simulink model "quadrotor_sim"  (Simulink 7.7)
settings: Solver=FixedStepDiscrete  StartTime=0.0  StopTime=120  FixedStep=1/50  RelTol=1e-3
undefined symbols (not defined in the file): alpha_IERA_IELA_IELA, bus_Environment, Kutta, R_IERA_RA_RA, Runge
libraries: UAVdesign_net x8
settings Model: Creator=Emanuel  LastModifiedBy=Emanuel
settings SFSimCC: SimCustomHeaderCode="#include \"cd_signals.h\""  SimUserSources=cd_signals.c

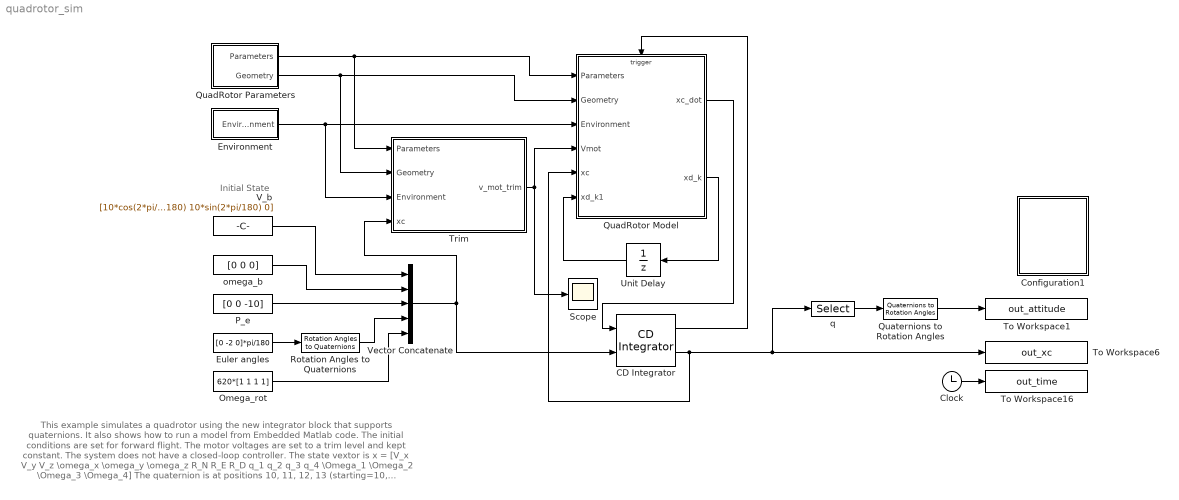
== system quadrotor_sim ==
  note: This example simulates a quadrotor using the new integrator block that supports quaternions. It also shows how to run a model from Embedded Matlab code.
      | The initial conditions are set for forward flight. The motor voltages are set to a trim level and kept constant. The system does not have a closed-loop controller.
      | The state vextor is x = [V_x V_y V_z   \omega_x \omega_y \omega_z    R_N R_E R_D    q_1 q_2 q_3 q_4    \Omega_1 \Omega_2 \Omega_3 \Omega_4]
      | The quaternion is at positions 10, 11, 12, 13 (starting=10, ending=13)
      | \Omega^{\bullet} is at positions 4, 5, 6
  note: Initial State
  CD Integrator : UAVdesign_net/Utilities/Continuous/CD Integrator  algorithm=Runge-Kutta  param_source=Discrete steps of the model  initial_time=0  final_time=10  reset_type=None  x0_source=External  x0=0  output_time=off  limit_output=off  upper_sat=inf  lower_sat=-inf  q_index=[10 13]  omega_dot_index=[4 6]  sample_time=-1
  Clock : Clock
  Configuration1 : Subsystem
      settings: OpenFcn=graphs_quadrotor_sim;
      mask Display: disp('Double-click\nto display\nthe\ngraphs')
  Environment : Subsystem  InitFcn=bus_Environment;
  Euler angles : Constant  Value=[0 -2 0]*pi/180
  Omega_rot : Constant  Value=620*[1 1 1 1]
  P_e : Constant  Value=[0 0 -10]
  QuadRotor Model : Subsystem
  QuadRotor Parameters : Subsystem  InitFcn=|  mask(HelicopterParameters){}
      | bus_PropellerParameters;    
      | bus_ElectricMotorParameters;
      | bus_GeometryParameters;     
      | bus_FuselageParameters;
      mask help:
      | Parameters for a helicopter.
      | Geometry, rotors, fuselage, fins.
      mask init:
      | set_param(gcb, 'LinkStatus', 'none');
      settings: OpenFcn=gui_QuadRotorParameters( 'Block', [get_param(gcb, 'Parent') '/' get_param(gcb, 'Name')]);
      mask Display:
      | port_label('output', 1, 'Parameters')
      | port_label('output', 2, 'Geometry')
  Quaternions to Rotation Angles : UAVdesign_net/Utilities/Axes/Quaternions to Rotation Angles  SystemSampleTime=-1
  Rotation Angles to Quaternions : UAVdesign_net/Utilities/Axes/Rotation Angles to Quaternions  SystemSampleTime=-1
  Scope : Scope
      settings: YMin=7.37  YMax=7.415
  To Workspace1 : ToWorkspace  VariableName=out_attitude  SampleTime=-1  SaveFormat=Array
  To Workspace16 : ToWorkspace  VariableName=out_time  SampleTime=-1  SaveFormat=Array
  To Workspace6 : ToWorkspace  VariableName=out_xc  SampleTime=-1  SaveFormat=Array
  Trim : Subsystem
  Unit Delay : UnitDelay  X0=[zeros(12,1); 1;1;1;1; zeros(7,1)]  SampleTime=-1
  V_b : Constant  Value=[10*cos(2*pi/180) 10*sin(2*pi/180) 0]
  Vector Concatenate : Concatenate  NumInputs=5  Mode=Vector
  omega_b : Constant  Value=[0 0 0]
  q : Selector  InputPortWidth=17  IndexOptions=Index vector (dialog)  Indices=[10:13]  OutputSizes=1
  wires:
  QuadRotor Model/2(xd_k) -> Unit Delay/1
  Unit Delay/1 -> QuadRotor Model/6(xd_k1)
  QuadRotor Model/1(xc_dot) -> CD Integrator/1
  CD Integrator/1 -> QuadRotor Model/Trigger
  CD Integrator/2 -> QuadRotor Model/5(xc), To Workspace6/1, q/1
  QuadRotor Parameters/1(Parameters) -> QuadRotor Model/1(Parameters), Trim/1(Parameters)
  QuadRotor Parameters/2(Geometry) -> QuadRotor Model/2(Geometry), Trim/2(Geometry)
  Environment/1(Environment) -> QuadRotor Model/3(Environment), Trim/3(Environment)
  Trim/1(v_mot_trim) -> QuadRotor Model/4(Vmot), Scope/1
  Clock/1 -> To Workspace16/1
  q/1 -> Quaternions to Rotation Angles/1
  Quaternions to Rotation Angles/1 -> To Workspace1/1
  Euler angles/1 -> Rotation Angles to Quaternions/1
  V_b/1 -> Vector Concatenate/1
  omega_b/1 -> Vector Concatenate/2
  P_e/1 -> Vector Concatenate/3
  Rotation Angles to Quaternions/1 -> Vector Concatenate/4
  Omega_rot/1 -> Vector Concatenate/5
  Vector Concatenate/1 -> CD Integrator/2, Trim/4(xc)

== system quadrotor_sim/Configuration1 ==

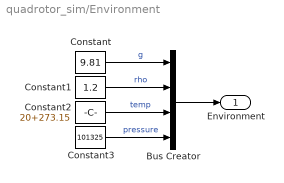
== system quadrotor_sim/Environment ==
  Bus Creator : BusCreator  NonVirtualBus=on
  Constant : Constant  Value=9.81
  Constant1 : Constant  Value=1.2
  Constant2 : Constant  Value=20+273.15
  Constant3 : Constant  Value=101325
  Environment : Outport
  wires:
  Constant3/1 -> Bus Creator/4  "pressure"
  Constant2/1 -> Bus Creator/3  "temp"
  Constant1/1 -> Bus Creator/2  "rho"
  Constant/1 -> Bus Creator/1  "g"
  Bus Creator/1 -> Environment/1

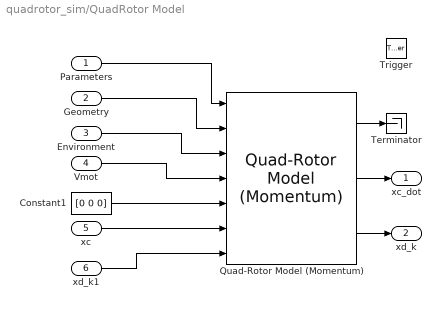
== system quadrotor_sim/QuadRotor Model ==
  Parameters : Inport
  Geometry : Inport  Port=2
  Environment : Inport  Port=3
  Vmot : Inport  Port=4
  xc : Inport  Port=5
  xd_k1 : Inport  Port=6
  Trigger : TriggerPort  TriggerType=function-call
  Constant1 : Constant  Value=[0 0 0]
  Quad-Rotor Model (Momentum) : UAVdesign_net/Vehicle Models/Quad-Rotor Model (Momentum)  SystemSampleTime=-1
  Terminator : Terminator
  xc_dot : Outport
  xd_k : Outport  Port=2
  wires:
  Geometry/1 -> Quad-Rotor Model (Momentum)/2
  xd_k1/1 -> Quad-Rotor Model (Momentum)/7
  xc/1 -> Quad-Rotor Model (Momentum)/6
  Environment/1 -> Quad-Rotor Model (Momentum)/3
  Parameters/1 -> Quad-Rotor Model (Momentum)/1
  Quad-Rotor Model (Momentum)/1 -> Terminator/1
  Constant1/1 -> Quad-Rotor Model (Momentum)/5
  Vmot/1 -> Quad-Rotor Model (Momentum)/4
  Quad-Rotor Model (Momentum)/3 -> xd_k/1
  Quad-Rotor Model (Momentum)/2 -> xc_dot/1

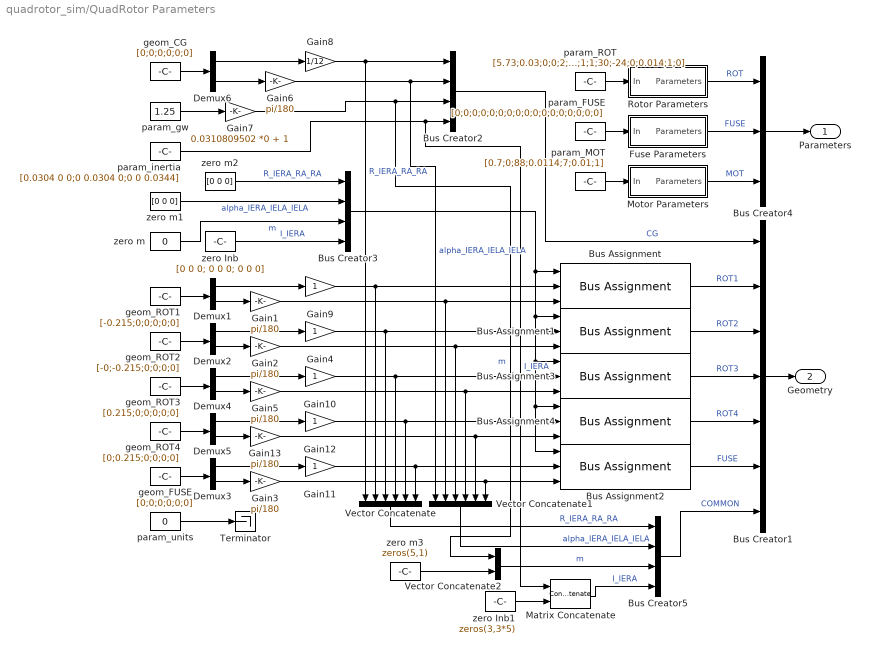
== system quadrotor_sim/QuadRotor Parameters ==
  Bus Assignment{,1..4} (5 alike) : BusAssignment  AssignedSignals=R_IERA_RA_RA,alpha_IERA_IELA_IELA
  Bus Creator1 : BusCreator  Inputs=7
  Bus Creator2 : BusCreator
  Bus Creator3 : BusCreator
  Bus Creator4 : BusCreator  Inputs=3
  Bus Creator5 : BusCreator
  Demux{1..6} (6 alike) : Demux  Outputs=2
  Fuse Parameters : Subsystem
  Gain{1..3,5..6,13} (6 alike) : Gain  Gain=pi/180
  Gain{4,9..12} (5 alike) : Gain
  Gain7 : Gain  Gain=0.0310809502 *0 + 1
  Gain8 : Gain  Gain=1/12
  Matrix Concatenate : Concatenate  Mode=Multidimensional array  ConcatenateDimension=2
  Motor Parameters : Subsystem
  Rotor Parameters : Subsystem
  Terminator : Terminator
  Vector Concatenate : Concatenate  NumInputs=6  Mode=Vector
  Vector Concatenate1 : Concatenate  NumInputs=6  Mode=Vector
  Vector Concatenate2 : Concatenate  Mode=Vector
  geom_CG : Constant  Value=[0;0;0;0;0;0]
  geom_FUSE : Constant  Value=[0;0;0;0;0;0]
  geom_ROT1 : Constant  Value=[-0.215;0;0;0;0;0]
  geom_ROT2 : Constant  Value=[-0;-0.215;0;0;0;0]
  geom_ROT3 : Constant  Value=[0.215;0;0;0;0;0]
  geom_ROT4 : Constant  Value=[0;0.215;0;0;0;0]
  param_FUSE : Constant  Value=[0;0;0;0;0;0;0;0;0;0;0;0;0;0;0;0;0]
  param_MOT : Constant  Value=[0.7;0;88;0.0114;7;0.01;1]
  param_ROT : Constant  Value=[5.73;0.03;0;0;2;0.127;0.016;0.95;1;1;30;-24;0;0.014;1;0]
  param_gw : Constant  Value=1.25
  param_inertia : Constant  Value=[0.0304 0 0;0 0.0304 0;0 0 0.0344]
  param_units : Constant  Value=0
  zero Inb : Constant  Value=[0 0 0; 0 0 0; 0 0 0]
  zero Inb1 : Constant  Value=zeros(3,3*5)
  zero m : Constant  Value=0
  zero m1 : Constant  Value=[0 0 0]
  zero m2 : Constant  Value=[0 0 0]
  zero m3 : Constant  Value=zeros(5,1)
  Parameters : Outport
  Geometry : Outport  Port=2
  wires:
  zero m3/1 -> Vector Concatenate2/2
  Vector Concatenate2/1 -> Bus Creator5/3  "m"
  Bus Creator1/1 -> Geometry/1
  Demux6/1 -> Gain8/1
  Demux6/2 -> Gain6/1
  param_gw/1 -> Gain7/1
  Demux1/1 -> Gain9/1
  Demux1/2 -> Gain1/1
  geom_ROT1/1 -> Demux1/1
  Demux3/1 -> Gain11/1
  Demux3/2 -> Gain3/1
  geom_FUSE/1 -> Demux3/1
  geom_CG/1 -> Demux6/1
  Bus Creator3/1 -> Bus Assignment/1, Bus Assignment1/1, Bus Assignment3/1, Bus Assignment2/1, Bus Assignment4/1
  Bus Creator4/1 -> Parameters/1
  param_ROT/1 -> Rotor Parameters/1(In)
  param_FUSE/1 -> Fuse Parameters/1(In)
  Gain1/1 -> Bus Assignment/3, Vector Concatenate1/2
  Gain3/1 -> Bus Assignment2/3, Vector Concatenate1/6
  Gain11/1 -> Bus Assignment2/2, Vector Concatenate/6
  Bus Assignment2/1 -> Bus Creator1/6  "FUSE"
  Bus Assignment/1 -> Bus Creator1/2  "ROT1"
  Bus Creator2/1 -> Bus Creator1/1  "CG"
  zero m2/1 -> Bus Creator3/1  "R_IERA_RA_RA"
  zero m1/1 -> Bus Creator3/2  "alpha_IERA_IELA_IELA"
  param_units/1 -> Terminator/1
  Rotor Parameters/1(Parameters) -> Bus Creator4/1  "ROT"
  Fuse Parameters/1(Parameters) -> Bus Creator4/2  "FUSE"
  Gain8/1 -> Bus Creator2/1, Vector Concatenate/1  "R_IERA_RA_RA"
  Gain6/1 -> Bus Creator2/2, Vector Concatenate1/1  "alpha_IERA_IELA_IELA"
  zero Inb/1 -> Bus Creator3/4  "I_IERA"
  zero m/1 -> Bus Creator3/3  "m"
  Gain7/1 -> Vector Concatenate2/1, Bus Creator2/3  "m"
  param_inertia/1 -> Bus Creator2/4, Matrix Concatenate/1  "I_IERA"
  Demux2/1 -> Gain4/1
  Demux2/2 -> Gain2/1
  Gain2/1 -> Bus Assignment1/3, Vector Concatenate1/3
  Gain4/1 -> Bus Assignment1/2, Vector Concatenate/3
  geom_ROT2/1 -> Demux2/1
  Gain9/1 -> Bus Assignment/2, Vector Concatenate/2
  Demux4/1 -> Gain10/1
  Demux4/2 -> Gain5/1
  Gain5/1 -> Bus Assignment3/3, Vector Concatenate1/4
  Gain10/1 -> Bus Assignment3/2, Vector Concatenate/4
  geom_ROT3/1 -> Demux4/1
  Demux5/1 -> Gain12/1
  Demux5/2 -> Gain13/1
  Gain13/1 -> Bus Assignment4/3, Vector Concatenate1/5
  Gain12/1 -> Bus Assignment4/2, Vector Concatenate/5
  geom_ROT4/1 -> Demux5/1
  Bus Assignment1/1 -> Bus Creator1/3  "ROT2"
  Bus Assignment3/1 -> Bus Creator1/4  "ROT3"
  Bus Assignment4/1 -> Bus Creator1/5  "ROT4"
  Bus Creator5/1 -> Bus Creator1/7  "COMMON"
  Vector Concatenate1/1 -> Bus Creator5/2  "alpha_IERA_IELA_IELA"
  Matrix Concatenate/1 -> Bus Creator5/4  "I_IERA"
  Vector Concatenate/1 -> Bus Creator5/1  "R_IERA_RA_RA"
  zero Inb1/1 -> Matrix Concatenate/2
  param_MOT/1 -> Motor Parameters/1(In)
  Motor Parameters/1(Parameters) -> Bus Creator4/3  "MOT"

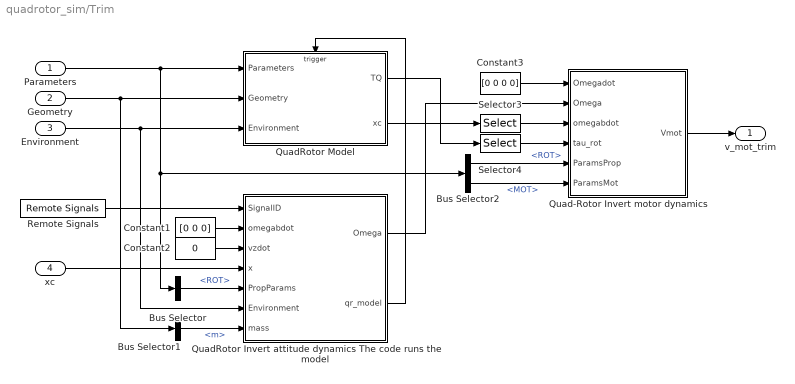
== system quadrotor_sim/Trim ==
  Parameters : Inport
  Geometry : Inport  Port=2
  Environment : Inport  Port=3
  xc : Inport  Port=4
  Bus Selector : BusSelector  OutputSignals=ROT
  Bus Selector1 : BusSelector  OutputSignals=CG.m
  Bus Selector2 : BusSelector  OutputSignals=ROT,MOT
  Constant1 : Constant  Value=[0 0 0]
  Constant2 : Constant  Value=0
  Constant3 : Constant  Value=[0 0 0 0]
  Quad-Rotor Invert motor dynamics : Stateflow chart  TreatAsAtomicUnit=on
  QuadRotor Invert attitude dynamics The code runs the model : Stateflow chart  TreatAsAtomicUnit=on
  QuadRotor Model : Subsystem
  Remote Signals : UAVdesign_net/Utilities/Continuous/Remote Signals  block_name='InvFM_Omega'  op_mode=Generate the signals ID  port_vector=[17 5*4+3]  sample_time=-1
  Selector3 : Selector  InputPortWidth=17  IndexOptions=Index vector (dialog)  Indices=[4:6]  OutputSizes=1
  Selector4 : Selector  InputPortWidth=8  IndexOptions=Index vector (dialog)  Indices=[2 4 6 8]  OutputSizes=1
  v_mot_trim : Outport
  wires:
  Parameters/1 -> QuadRotor Model/1(Parameters), Bus Selector/1, Bus Selector2/1
  Geometry/1 -> QuadRotor Model/2(Geometry), Bus Selector1/1
  Environment/1 -> QuadRotor Model/3(Environment), QuadRotor Invert attitude dynamics The code runs the model/6(Environment)
  Remote Signals/1 -> QuadRotor Invert attitude dynamics The code runs the model/1(SignalID)
  QuadRotor Invert attitude dynamics The code runs the model/2(qr_model) -> QuadRotor Model/Trigger
  xc/1 -> QuadRotor Invert attitude dynamics The code runs the model/4(x)
  Bus Selector/1 -> QuadRotor Invert attitude dynamics The code runs the model/5(PropParams)  "<ROT>"
  Bus Selector1/1 -> QuadRotor Invert attitude dynamics The code runs the model/7(mass)  "<m>"
  Constant1/1 -> QuadRotor Invert attitude dynamics The code runs the model/2(omegabdot)
  Constant2/1 -> QuadRotor Invert attitude dynamics The code runs the model/3(vzdot)
  Selector3/1 -> Quad-Rotor Invert motor dynamics/3(omegabdot)
  Selector4/1 -> Quad-Rotor Invert motor dynamics/4(tau_rot)
  Bus Selector2/1 -> Quad-Rotor Invert motor dynamics/5(ParamsProp)  "<ROT>"
  Bus Selector2/2 -> Quad-Rotor Invert motor dynamics/6(ParamsMot)  "<MOT>"
  Constant3/1 -> Quad-Rotor Invert motor dynamics/1(Omegadot)
  QuadRotor Invert attitude dynamics The code runs the model/1(Omega) -> Quad-Rotor Invert motor dynamics/2(Omega)
  QuadRotor Model/1(TQ) -> Selector4/1
  QuadRotor Model/2(xc) -> Selector3/1
  Quad-Rotor Invert motor dynamics/1(Vmot) -> v_mot_trim/1

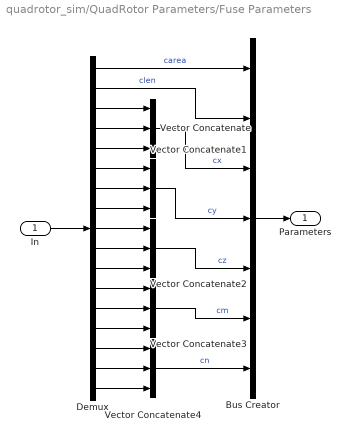
== system quadrotor_sim/QuadRotor Parameters/Fuse Parameters ==
  In : Inport
  Bus Creator : BusCreator  Inputs=7  OutDataTypeStr=Bus: FuselageParameters  NonVirtualBus=on
  Demux : Demux  Outputs=17
  Vector Concatenate{,1..4} (5 alike) : Concatenate  NumInputs=3  Mode=Vector
  Parameters : Outport  OutDataTypeStr=Bus: FuselageParameters
  wires:
  Demux/1 -> Bus Creator/1  "carea"
  Bus Creator/1 -> Parameters/1
  In/1 -> Demux/1
  Demux/2 -> Bus Creator/2  "clen"
  Demux/3 -> Vector Concatenate/1
  Demux/4 -> Vector Concatenate/2
  Demux/5 -> Vector Concatenate/3
  Vector Concatenate/1 -> Bus Creator/3  "cx"
  Demux/6 -> Vector Concatenate1/1
  Demux/7 -> Vector Concatenate1/2
  Demux/8 -> Vector Concatenate1/3
  Vector Concatenate1/1 -> Bus Creator/4  "cy"
  Demux/9 -> Vector Concatenate2/1
  Demux/10 -> Vector Concatenate2/2
  Demux/11 -> Vector Concatenate2/3
  Vector Concatenate2/1 -> Bus Creator/5  "cz"
  Demux/12 -> Vector Concatenate3/1
  Demux/13 -> Vector Concatenate3/2
  Demux/14 -> Vector Concatenate3/3
  Demux/15 -> Vector Concatenate4/1
  Demux/16 -> Vector Concatenate4/2
  Demux/17 -> Vector Concatenate4/3
  Vector Concatenate3/1 -> Bus Creator/6  "cm"
  Vector Concatenate4/1 -> Bus Creator/7  "cn"

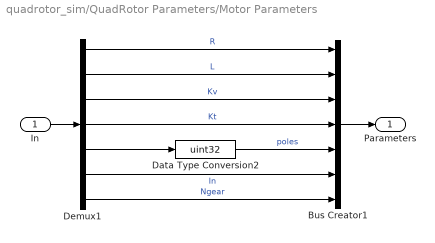
== system quadrotor_sim/QuadRotor Parameters/Motor Parameters ==
  In : Inport
  Bus Creator1 : BusCreator  Inputs=7  NonVirtualBus=on
  Data Type Conversion2 : DataTypeConversion  OutDataTypeStr=uint32  RndMeth=Nearest
  Demux1 : Demux  Outputs=7
  Parameters : Outport
  wires:
  In/1 -> Demux1/1
  Bus Creator1/1 -> Parameters/1
  Demux1/1 -> Bus Creator1/1  "R"
  Demux1/2 -> Bus Creator1/2  "L"
  Demux1/3 -> Bus Creator1/3  "Kv"
  Demux1/4 -> Bus Creator1/4  "Kt"
  Demux1/5 -> Data Type Conversion2/1
  Data Type Conversion2/1 -> Bus Creator1/5  "poles"
  Demux1/6 -> Bus Creator1/6  "In"
  Demux1/7 -> Bus Creator1/7  "Ngear"

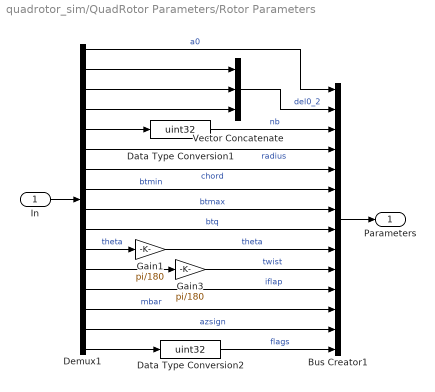
== system quadrotor_sim/QuadRotor Parameters/Rotor Parameters ==
  In : Inport
  Bus Creator1 : BusCreator  Inputs=14  NonVirtualBus=on
  Data Type Conversion1 : DataTypeConversion  OutDataTypeStr=uint32  RndMeth=Nearest
  Data Type Conversion2 : DataTypeConversion  OutDataTypeStr=uint32  RndMeth=Nearest
  Demux1 : Demux  Outputs=16
  Gain1 : Gain  Gain=pi/180
  Gain3 : Gain  Gain=pi/180
  Vector Concatenate : Concatenate  NumInputs=3  Mode=Vector
  Parameters : Outport
  wires:
  Demux1/15 -> Bus Creator1/13  "azsign"
  Demux1/14 -> Bus Creator1/12  "mbar"
  Demux1/13 -> Bus Creator1/11  "iflap"
  Demux1/9 -> Bus Creator1/7  "btmax"
  Demux1/1 -> Bus Creator1/1  "a0"
  Bus Creator1/1 -> Parameters/1
  Demux1/4 -> Vector Concatenate/3
  Demux1/3 -> Vector Concatenate/2
  Demux1/2 -> Vector Concatenate/1
  In/1 -> Demux1/1
  Data Type Conversion1/1 -> Bus Creator1/3  "nb"
  Demux1/5 -> Data Type Conversion1/1
  Demux1/6 -> Bus Creator1/4  "radius"
  Demux1/7 -> Bus Creator1/5  "chord"
  Demux1/8 -> Bus Creator1/6  "btmin"
  Demux1/12 -> Gain3/1
  Demux1/10 -> Bus Creator1/8  "btq"
  Demux1/11 -> Gain1/1  "theta"
  Gain1/1 -> Bus Creator1/9  "theta"
  Vector Concatenate/1 -> Bus Creator1/2  "del0_2"
  Gain3/1 -> Bus Creator1/10  "twist"
  Demux1/16 -> Data Type Conversion2/1
  Data Type Conversion2/1 -> Bus Creator1/14  "flags"

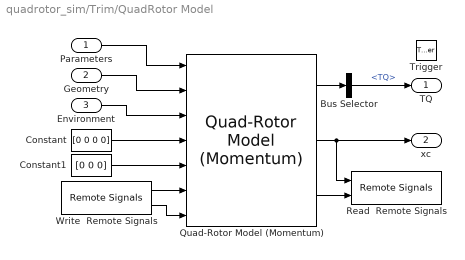
== system quadrotor_sim/Trim/QuadRotor Model ==
  Parameters : Inport
  Geometry : Inport  Port=2
  Environment : Inport  Port=3
  Trigger : TriggerPort  TriggerType=function-call
  Bus Selector : BusSelector  OutputSignals=TQ
  Constant : Constant  Value=[0 0 0 0]
  Constant1 : Constant  Value=[0 0 0]
  Quad-Rotor Model (Momentum) : UAVdesign_net/Vehicle Models/Quad-Rotor Model (Momentum)  SystemSampleTime=-1
  Read  Remote Signals : UAVdesign_net/Utilities/Continuous/Remote Signals  block_name='InvFM_Omega'  op_mode=Read the output  port_vector=[17 5*4+3]  sample_time=-1
  Write  Remote Signals : UAVdesign_net/Utilities/Continuous/Remote Signals  block_name='InvFM_Omega'  op_mode=Write the input  port_vector=[17 5*4+3]  sample_time=-1
  TQ : Outport
  xc : Outport  Port=2
  wires:
  Quad-Rotor Model (Momentum)/2 -> Read  Remote Signals/1, xc/1
  Quad-Rotor Model (Momentum)/3 -> Read  Remote Signals/2
  Constant/1 -> Quad-Rotor Model (Momentum)/4
  Constant1/1 -> Quad-Rotor Model (Momentum)/5
  Write  Remote Signals/1 -> Quad-Rotor Model (Momentum)/6
  Write  Remote Signals/2 -> Quad-Rotor Model (Momentum)/7
  Quad-Rotor Model (Momentum)/1 -> Bus Selector/1
  Parameters/1 -> Quad-Rotor Model (Momentum)/1
  Geometry/1 -> Quad-Rotor Model (Momentum)/2
  Environment/1 -> Quad-Rotor Model (Momentum)/3
  Bus Selector/1 -> TQ/1  "<TQ>"

== matlab function Trim/QuadRotor Invert attitude dynamics The code runs the model ==
  data: SignalID input double; omegabdot input double; vzdot input double; Omega output double; x input double; PropParams input Bus: PropellerParameters size=1; Environment input Bus: Environment size=1; mass input double
  events: qr_model output FUNCTION_CALL_EVENT
function Omega = qinv_att(SignalID, omegabdot, vzdot, x, PropParams, Environment, mass)

persistent prev_data

if isempty(prev_data)


% Find the approximative value of omega_rot that generates the requested vzdot
% It will be later used in the trim algorithm as a start value
% vzdot includes the effect of g (e.g. vzdot = 0 means hover)
rho    = Environment.rho;
radius = PropParams.radius;
nb     = double(PropParams.nb);
chord  = PropParams.chord;
a0     = PropParams.a0;
theta0 = PropParams.theta;
twist  = PropParams.twist;

q_ag   = [0; 0; 0; Environment.g];
q_ag   = qprod(x(10:13).*[1; -1; -1; -1], q_ag);
q_ag   = qprod(q_ag, x(10:13));

Fz_rot = abs(vzdot-q_ag(4))*mass/4;
fact1  = rho*radius*nb*chord*a0;
delta  = fact1^2 / (32*rho*pi);
delta  = delta + 2*fact1*radius^2*(1/3*theta0+1/4*twist);
omega_rot = fact1 / (4*sqrt(2*rho*pi)) + sqrt(delta);
omega_rot = omega_rot * sqrt(Fz_rot);
omega_rot = omega_rot / (fact1*radius^2*(1/3*theta0+1/4*twist));

Nin  = 4;
Nout = 4;
pos_in  = [14:17];
pos_out = [4:6 3];
du      = [1; 1; 1; 1]*pi;
jac  = zeros(Nout, Nin);
u_temp = zeros(17,1);
y_temp = zeros(17,1);
u0   = x;
u0(pos_in) = omega_rot*ones(Nin, 1);
xd = zeros(5*4+3, 1);
xd(13:16) = [1; 1; 1; 1];
y0 = [omegabdot; vzdot];

% find xd
cd_set_signal(SignalID, 0, u0);
cd_set_signal(SignalID, 1, xd);
qr_model;
xd = cd_get_signal(SignalID, 1, length(xd));

% Newton-Raphson iteration
for i=1:3
    cd_set_signal(SignalID, 1, xd);
    
    % find Jacobian
    index_in  = 1;
    while index_in <= Nin
        u_temp = u0;
        u_temp(pos_in(index_in)) = u_temp(pos_in(index_in)) + du(index_in);

        cd_set_signal(SignalID, 0, u_temp);
        qr_model;
        y_temp = cd_get_signal(SignalID, 0, length(y_temp));
        jac(:, index_in) = y_temp(pos_out);
        index_in = index_in + 1;
    end
    cd_set_signal(SignalID, 0, u0);
    qr_model;
    y_temp = cd_get_signal(SignalID, 0, length(y_temp));
    xd = cd_get_signal(SignalID, 1, length(xd));

    index_out = 1;
    while index_out <= Nout
        jac(index_out, :) = jac(index_out, :) - y_temp(pos_out(index_out));
        index_out = index_out + 1;
    end
    index_in = 1;
    while index_in <= Nin
        jac(:,index_in) = jac(:,index_in) / du(index_in);
        index_in = index_in + 1;
    end
    
    % find next u0
    du0 = -inv(jac)*(y_temp(pos_out)-y0);
    u0(pos_in) = u0(pos_in) + du0;
    
    % find new xd
    cd_set_signal(SignalID, 0, u0);
    cd_set_signal(SignalID, 1, xd);
    qr_model;
    y_temp = cd_get_signal(SignalID, 0, length(y_temp));
    xd = cd_get_signal(SignalID, 1, length(xd));
end
prev_data = u0(pos_in);

else
    % do nothing
end
Omega = prev_data;

function qr = qprod(q, r)
qr = zeros(4,1);
qr(1) = q(1)*r(1) - q(2)*r(2) - q(3)*r(3) - q(4)*r(4);
qr(2) = q(2)*r(1) + q(1)*r(2) - q(4)*r(3) + q(3)*r(4);
qr(3) = q(3)*r(1) + q(4)*r(2) + q(1)*r(3) - q(2)*r(4);
qr(4) = q(4)*r(1) - q(3)*r(2) + q(2)*r(3) + q(1)*r(4);

== matlab function Trim/Quad-Rotor Invert motor dynamics ==
  data: Omegadot input double; Omega input double; omegabdot input double; tau_rot input double; Vmot output double; ParamsProp input Bus: PropellerParameters size=1; ParamsMot input Bus: ElectricMotorParameters size=1
function Vmot = qrinv_mot(Omegadot, Omega, omegabdot, tau_rot, ParamsProp, ParamsMot)

if ParamsProp.iflap
    iflap = ParamsProp.iflap;
else
    iflap = ParamsProp.mbar * ParamsProp.radius^3 / 3;
end


Vmot = double(ParamsProp.nb)*iflap * (Omegadot + omegabdot(3)*ParamsProp.azsign*[1; -1; 1; -1]) + tau_rot;
Vmot = Vmot * ParamsMot.R/ParamsMot.Kt;
Vmot = Vmot + 1/ParamsMot.Kv*Omega;
